simulink subsystem "Physical_Plant_Hardware"  (R2025b)
settings: Solver=VariableStepAuto  StartTime=0.0  StopTime=10.0  RelTol=1e-3
undefined symbols (not defined in the file or in its folder): Ion, Lithium
libraries: spsGroundLib x4, spsBatteryLib x2, spsIdealSwitchLib x2, spsUniversalBridgeLib x2, spsCurrentMeasurementLib x1, spsLinearTransformerLib x1, spsSeriesRLCBranchLib x1, spsSeriesRLCLoadLib x1, spsVoltageMeasurementLib x1
settings Model: Creator=admin  LastModifiedBy=admin

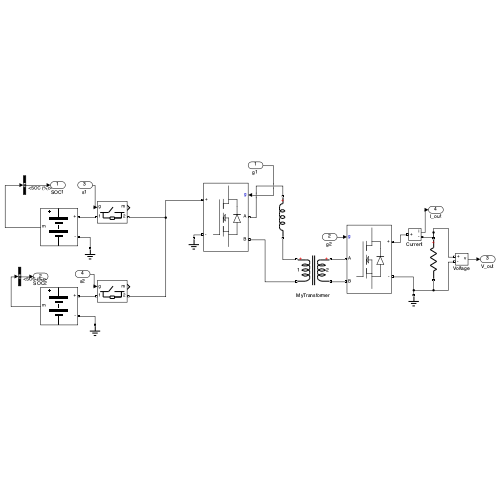
[thumbnail: Simulink's stored preview of the top-level diagram]
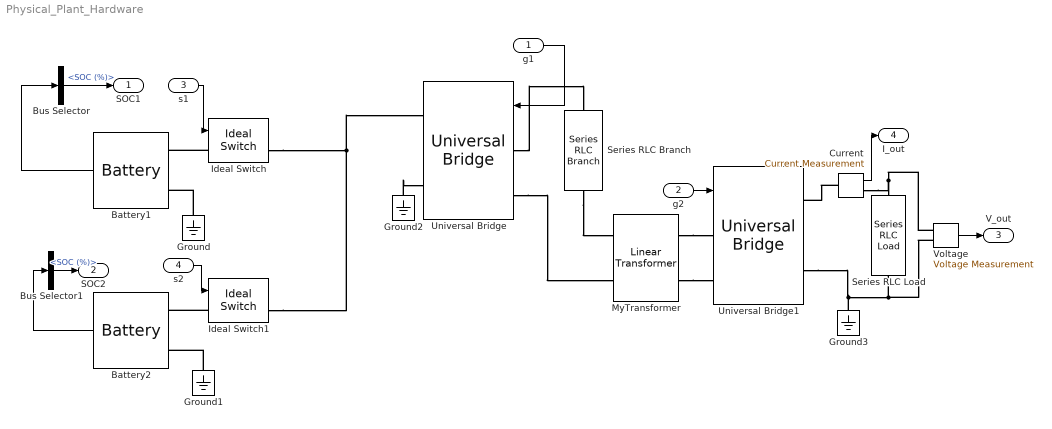
== system Physical_Plant_Hardware ==
  g1 : Inport
  g2 : Inport  Port=2
  s1 : Inport  Port=3
  s2 : Inport  Port=4
  Battery1 : spsBatteryLib/Battery  BatType=Lithium-Ion  NomV=50  NomQ=40  SOC=80  Batt_Tr=1  PresetModel=on  MaxQ=40  MinV=37.5  FullV=58.1994  Dis_rate=17.3913  R=0.0125  Normal_OP=36.1739  expZone="[54.0193      1.96522]"
  Battery2 : spsBatteryLib/Battery  BatType=Lithium-Ion  NomV=50  NomQ=40  SOC=70  Batt_Tr=1  PresetModel=on  MaxQ=40  MinV=37.5  FullV=58.1994  Dis_rate=17.3913  R=0.0125  Normal_OP=36.1739  expZone="[54.0193      1.96522]"
  Bus Selector : BusSelector  OutputSignals=SOC (%)
  Bus Selector1 : BusSelector  OutputSignals=SOC (%)
  Current : spsCurrentMeasurementLib/Current Measurement  PhasorSimulation=off  OutputType=Complex  PSBequivalent=0
  Ground{,1..3} (4 alike) : spsGroundLib/Ground  LConnTagsString=a
  Ideal Switch : spsIdealSwitchLib/Ideal Switch  Ron=0.001  Lon=0  IC=0  Rs=1e5  Cs=inf  Measurements=on
  Ideal Switch1 : spsIdealSwitchLib/Ideal Switch  Ron=0.001  Lon=0  IC=0  Rs=1e5  Cs=inf  Measurements=on
  MyTransformer : spsLinearTransformerLib/Linear Transformer  UNITS=SI  NominalPower=[ 2000 20000 ]  winding1=[ 50 0.002 0]  winding2=[50 0.002 0]  ThreeWindings=off  winding3=[3.15e+05 0.7938 0.084225]  RmLm=[5000 1]  Measurements=None  DataType=on
  Series RLC Branch : spsSeriesRLCBranchLib/Series RLC Branch  LConnTagsString=__new0  RConnTagsString=__new0  BranchType=L  Resistance=1  Inductance=20e-6  SetiL0=off  InitialCurrent=0  Capacitance=1e-6  Setx0=off  InitialVoltage=0  Measurements=None
  Series RLC Load : spsSeriesRLCLoadLib/Series RLC Load  LConnTagsString=a  RConnTagsString=__new0  NominalVoltage=50  NominalFrequency=0  ActivePower=2000  InductivePower=0  CapacitivePower=0  Setx0=off  InitialVoltage=0  SetiL0=off  InitialCurrent=0  Measurements=None  LoadType=constant Z
  Universal Bridge : spsUniversalBridgeLib/Universal Bridge  Arms=2  SnubberResistance=1e5  SnubberCapacitance=inf  Device=MOSFET / Diodes  Ron=1e-3  Lon=0  ForwardVoltages="[  0  0  ]"  ForwardVoltage=0  GTOparameters=[ 10e-6 , 20e-6 ]  IGBTparameters=[ 1e-6 , 2e-6 ]  Measurements=None  Measurements_2=None  converterType=Rectifier
  Universal Bridge1 : spsUniversalBridgeLib/Universal Bridge  Arms=2  SnubberResistance=1e5  SnubberCapacitance=inf  Device=MOSFET / Diodes  Ron=1e-3  Lon=0  ForwardVoltages="[  0  0  ]"  ForwardVoltage=0  GTOparameters=[ 10e-6 , 20e-6 ]  IGBTparameters=[ 1e-6 , 2e-6 ]  Measurements=None  Measurements_2=None  converterType=Rectifier
  Voltage : spsVoltageMeasurementLib/Voltage Measurement  PhasorSimulation=off  OutputType=Complex  PSBequivalent=0
  SOC1 : Outport
  SOC2 : Outport  Port=2
  V_out : Outport  Port=3
  I_out : Outport  Port=4
  wires:
  Battery1/1 -> Bus Selector/1
  Battery2/1 -> Bus Selector1/1
  Bus Selector/1 -> SOC1/1  "<SOC (%)>"
  Bus Selector1/1 -> SOC2/1  "<SOC (%)>"
  Voltage/1 -> V_out/1
  Current/1 -> I_out/1
  g1/1 -> Universal Bridge/1
  g2/1 -> Universal Bridge1/1
  s1/1 -> Ideal Switch/1
  s2/1 -> Ideal Switch1/1
  connections:
  Voltage/LConn1 -- Current/RConn1 -- Series RLC Load/LConn1
  Universal Bridge1/RConn2 -- Ground3/LConn1 -- Voltage/LConn2 -- Series RLC Load/RConn1
  Universal Bridge/LConn1 -- Series RLC Branch/LConn1
  Series RLC Branch/RConn1 -- MyTransformer/LConn1
  Universal Bridge/LConn2 -- MyTransformer/LConn2
  MyTransformer/RConn1 -- Universal Bridge1/LConn1
  MyTransformer/RConn2 -- Universal Bridge1/LConn2
  Ground1/LConn1 -- Battery2/LConn2
  Ground/LConn1 -- Battery1/LConn2
  Ground2/LConn1 -- Universal Bridge/RConn2
  Ideal Switch/LConn1 -- Battery1/LConn1
  Ideal Switch/RConn1 -- Ideal Switch1/RConn1 -- Universal Bridge/RConn1
  Ideal Switch1/LConn1 -- Battery2/LConn1
  Current/LConn1 -- Universal Bridge1/RConn1
